simulink model "PID_Cdelta_U"  (R2019b)
settings: Solver=ode4  StartTime=0.0  StopTime=inf  FixedStep=0.05  RelTol=1e-3
InitFcn:
  | initModelParam;
  | SetWaypoints;
values from neighbouring files (symbols this model uses):
  Angsave = zeros(0, WPNum - 1)    [SetWaypoints.m]
  Deltah = 5    [reload.m]
  Deltav = 3    [reload.m]
  P0 = [0,0,0]    [SetWaypoints.m]
  rh = 0.005    [reload.m]
  rv = 0.003    [reload.m]
  Waypoints = [ ... (first row only)    [SetWaypoints.m]
  WPNum = 5    [SetWaypoints.m]
undefined symbols (not defined in the file or in its folder): DiscIntNeverNeededParam
libraries: simulink x3, vrlib x1
settings Model: Creator=53549  LastModifiedBy=51948
settings DataIOCC: ExternalInput=[]  ReturnWorkspaceOutputs=off  OutputSaveName=simOut
settings DebuggingCC: ArithmeticOperatorsInVariantConditions=warning
settings SFSimCC: SimUseLocalCustomCode=off  CustomCodeUndefinedFunction=UseInterfaceOnly
settings RTWCC: RTWUseLocalCustomCode=off
settings CodeAppCC: StateflowObjectComments=on

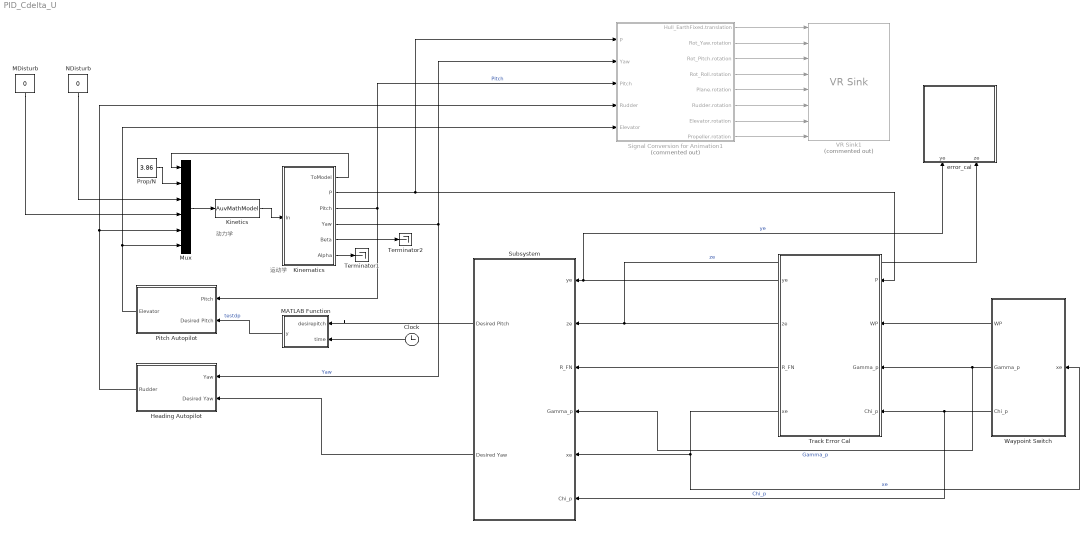
== system PID_Cdelta_U ==
  note: 运动学
  note: 动力学
  Clock : Clock
  Heading Autopilot : Subsystem  mask{kp=2, ki=0, kd=1.5, lambda=0.6, eta=30, epsilon=10, alpha=0.6, Modc=0}
      mask prompts: lambda "滑模表面斜率"; eta "控制增益"; epsilon "防抖动项"; alpha "filter coefficient"; Modc "大于0PID，等于0SMC"
      mask DialogControl DescGroupVar Prompt: Heading Autopilot
      mask DialogControl DescTextVar Prompt: 设置PID增益。
      mask DialogControl ParameterGroupVar Prompt: PID Parameter
  Kinematics : Subsystem  mask{x0=0, y0=0, z0=0.2, pitch0=-10, yaw0=45, u0=0.6, waveAmplitude=[0.2,0.3, 0.05], waveFrequency=[0.1, 0.15,0.2], deR=0.85}
      mask prompts: x0 "Initiral x"; y0 "Initiral y"; z0 "Initiral z"; pitch0 "Initial pitch [Deg]"; yaw0 "Initial yaw [Deg]"; u0 "Initial velocity [m/s]"; deR "decayRate"
      mask init:
      | waveAmplitude = str2num(get_param(gcb, 'waveAmplitude'));
      | waveFrequency = str2num(get_param(gcb, 'waveFrequency'));
      mask DialogControl DescGroupVar Prompt: Kinematics
      mask DialogControl DescTextVar Prompt: Set kinematics information: AMV initial state, flow interference, etc
      mask DialogControl ParameterGroupVar Prompt: Initial state
      mask DialogControl Container3 Prompt: Flow
  Kinetics : MATLABFcn  MATLABFcn=AuvMathModel  OutputDimensions=6  OutputSignalType=real
  MATLAB Function : MATLAB Function  TreatAsAtomicUnit=on
  MDisturb : Constant  Value=0
  Mux : Mux  Inputs=6
  NDisturb : Constant  Value=0
  Pitch Autopilot : Subsystem  mask{kp=3, ki=0.5, kd=1.5, lambda=0.6, eta=30, epsilon=10}
      mask prompts: lambda "滑模表面斜率"; eta "增大控制增益"; epsilon "减小防抖动项"
      mask DialogControl DescGroupVar Prompt: Pitch Autopilot
      mask DialogControl DescTextVar Prompt: 设置PID控制增益。
      mask DialogControl ParameterGroupVar Prompt: PID Parameter
  Prop/N : Constant  Value=3.86
  Signal Conversion for Animation1 : Subsystem  Commented=on
  Subsystem : Subsystem  mask{Deltah=Deltah, Deltav=Deltav, miuc=10, rh=rh, rv=rv}
      mask prompts: Deltah "水平面前视距离"; Deltav "垂直面前视距离"; miuc "极小正常数"; rh "βc自适应增益"; rv "αc自适应增益"
  Terminator1 : Terminator
  Terminator2 : Terminator
  Track Error Cal : MATLAB Function  TreatAsAtomicUnit=on
  VR Sink1 : vrlib/VR Sink  Commented=on  InstantiateOnLoad=on  SampleTime=0.1  ViewEnable=on  RemoteChange=off  RemoteView=off  FieldsWritten=NED.translation.3.1.1.double#RotYaw.rotation.4.1.1.double#RotPitch.rotation.4.1.1.double#RotRoll.rotation.4.1.1.double#Plane.rotation.4.1.1.double#Rudder.rotation.4.1.1.double#Elevator.rotation.4.1.1.double#Rotatation.rotation.4.1.1.double  WorldFileName=SubMarine.wrl  AutoView=on  VideoDimensions=[]  AllowVariableSize=off
      settings: SourceProductName=Simulink
  Waypoint Switch : Subsystem  mask{WP=Waypoints, Angsave=Angsave, WPNum=WPNum}
      mask prompts: WP "航点序列"; Angsave "航点夹角"; WPNum "航点个数"
      mask DialogControl DescGroupVar Prompt: 航点设置
      mask DialogControl DescTextVar Prompt: 设置航点序列和个数
  error_cal : Subsystem
  wires:
  Kinetics/1 -> Kinematics/1(In)
  Mux/1 -> Kinetics/1
  Kinematics/4(Yaw) -> Signal Conversion for Animation1/2(Yaw), Heading Autopilot/1(Yaw)  "Yaw"
  Kinematics/1(ToModel) -> Mux/1
  Prop/N/1 -> Mux/2
  NDisturb/1 -> Mux/3
  Track Error Cal/4(xe) -> Waypoint Switch/1(xe), Subsystem/5(xe)  "xe"
  Waypoint Switch/2(Gamma_p) -> Track Error Cal/3(Gamma_p), Subsystem/4(Gamma_p)  "Gamma_p"
  MDisturb/1 -> Mux/4
  Kinematics/2(P) -> Signal Conversion for Animation1/1(P), Track Error Cal/1(P)
  Kinematics/3(Pitch) -> Signal Conversion for Animation1/3(Pitch), Pitch Autopilot/1(Pitch)  "Pitch"
  Waypoint Switch/3(Chi_p) -> Track Error Cal/4(Chi_p), Subsystem/6(Chi_p)  "Chi_p"
  Waypoint Switch/1(WP) -> Track Error Cal/2(WP)
  Heading Autopilot/1(Rudder) -> Mux/5, Signal Conversion for Animation1/4(Rudder)
  Pitch Autopilot/1(Elevator) -> Signal Conversion for Animation1/5(Elevator), Mux/6
  Signal Conversion for Animation1/1(Hull_EarthFixed.translation) -> VR Sink1/1
  Signal Conversion for Animation1/2(Rot_Yaw.rotation) -> VR Sink1/2
  Signal Conversion for Animation1/3(Rot_Pitch.rotation) -> VR Sink1/3
  Signal Conversion for Animation1/4(Rot_Roll.rotation) -> VR Sink1/4
  Signal Conversion for Animation1/5(Plane.rotation) -> VR Sink1/5
  Signal Conversion for Animation1/8(Propeller.rotation) -> VR Sink1/8
  Signal Conversion for Animation1/6(Rudder.rotation) -> VR Sink1/6
  Signal Conversion for Animation1/7(Elevator.rotation) -> VR Sink1/7
  Subsystem/1(Desired Pitch) -> MATLAB Function/1(desirepitch)
  Subsystem/2(Desired Yaw) -> Heading Autopilot/2(Desired Yaw)
  Track Error Cal/1(ye) -> error_cal/1(ye), Subsystem/1(ye)  "ye"
  Track Error Cal/2(ze) -> error_cal/2(ze), Subsystem/2(ze)  "ze"
  Track Error Cal/3(R_FN) -> Subsystem/3(R_FN)
  Kinematics/6(Alpha) -> Terminator1/1
  Kinematics/5(Beta) -> Terminator2/1
  Clock/1 -> MATLAB Function/2(time)
  MATLAB Function/1(y) -> Pitch Autopilot/2(Desired Pitch)  "testdp"

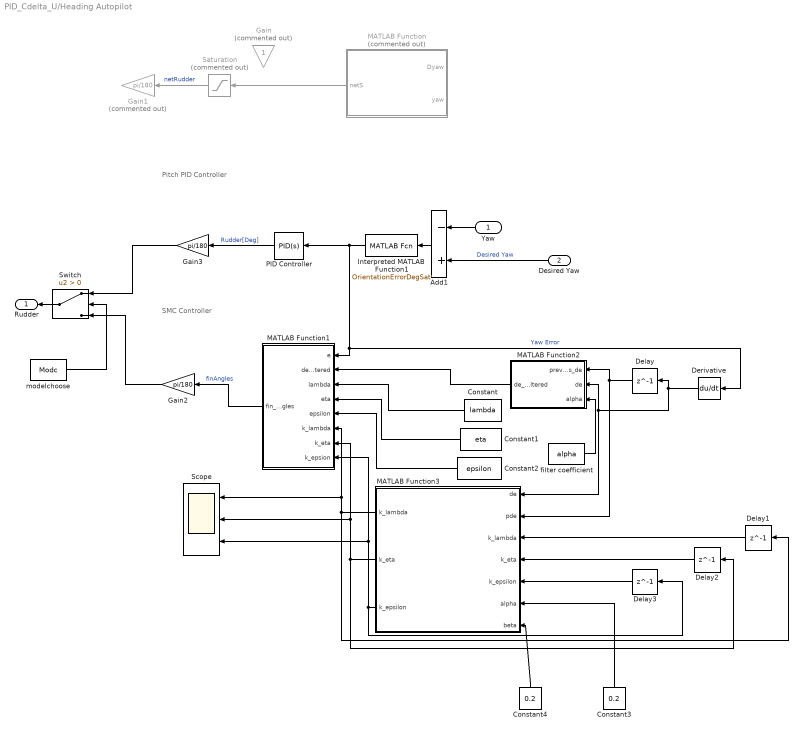
== system PID_Cdelta_U/Heading Autopilot ==
  note: SMC Controller
  note: Pitch PID Controller
  Yaw : Inport
  Desired Yaw : Inport  Port=2
  Add1 : Sum  Inputs=-+
  Constant : Constant  Value=lambda
  Constant1 : Constant  Value=eta
  Constant2 : Constant  Value=epsilon
  Constant3 : Constant  Value=0.2
  Constant4 : Constant  Value=0.2
  Delay{,1..3} (4 alike) : Delay  DelayLength=1
  Derivative : Derivative
  Gain : Gain  Commented=on
  Gain1 : Gain  Commented=on  Gain=pi/180
  Gain2 : Gain  Gain=pi/180
  Gain3 : Gain  Gain=pi/180
  Interpreted MATLAB Function1 : MATLABFcn  MATLABFcn=OrientationErrorDegSat  OutputDimensions=1
  MATLAB Function : MATLAB Function  Commented=on  TreatAsAtomicUnit=on  SystemSampleTime=0.05
  MATLAB Function1 : MATLAB Function  TreatAsAtomicUnit=on
  MATLAB Function2 : MATLAB Function  TreatAsAtomicUnit=on
  MATLAB Function3 : MATLAB Function  TreatAsAtomicUnit=on
  PID Controller : simulink/Continuous/PID Controller  Controller=PID  Form=Parallel  TimeDomain=Continuous-time  SampleTime=-1  IntegratorMethod=Forward Euler  FilterMethod=Forward Euler  ControllerParametersSource=internal  P=kp  I=ki  D=kd  UseFilter=on  N=10  TunerSelectOption=Transfer Function Based (PID Tuner App)  InitialConditionSource=internal  InitialConditionForIntegrator=0  InitialConditionForFilter=0  DifferentiatorICPrevScaledInput=0  ExternalReset=none  TrackingMode=off  Kt=1  LimitOutput=on  UpperSaturationLimit=30  LowerSaturationLimit=-30  LinearizeAsGain=on  AntiWindupMode=none  Kb=1  POutMin=[]  POutMax=[]  IOutMin=[]  IOutMax=[]  DOutMin=[]  DOutMax=[]  NOutMin=[]  NOutMax=[]  SumOutMin=[]  SumOutMax=[]  SaturationOutMin=[]  SaturationOutMax=[]  PParamMin=[]  PParamMax=[]  IParamMin=[]  IParamMax=[]  DParamMin=[]  DParamMax=[]  NParamMin=[]  NParamMax=[]  KbParamMin=[]  KbParamMax=[]  KtParamMin=[]  KtParamMax=[]  KbOutMin=[]  KbOutMax=[]  KtOutMin=[]  KtOutMax=[]  IntegratorOutMin=[]  IntegratorOutMax=[]  FilterOutMin=[]  FilterOutMax=[]  SumI1OutMin=[]  SumI1OutMax=[]  SumI2OutMin=[]  SumI2OutMax=[]  SumI3OutMin=[]  SumI3OutMax=[]  SumI4OutMin=[]  SumI4OutMax=[]  SumDOutMin=[]  SumDOutMax=[]  DifferentiatorOutMin=[]  DifferentiatorOutMax=[]  FilterDiffOutCoefMin=[]  FilterDiffOutCoefMax=[]  ReciprocalOutMin=[]  ReciprocalOutMax=[]  SumDenOutMin=[]  SumDenOutMax=[]  SumNumOutMin=[]  SumNumOutMax=[]  DivideOutMin=[]  DivideOutMax=[]  IntegratorContinuousStateAttributes=''  IntegratorStateMustResolveToSignalObject=off  IntegratorRTWStateStorageClass=Auto  FilterContinuousStateAttributes=''  FilterStateMustResolveToSignalObject=off  FilterRTWStateStorageClass=Auto  ParallelPVariant=InternalParameters  IdealPVariant=Disabled  IVariant=InternalParameters  DVariant=InternalParameters  IntegratorVariant=Continuous  SatVariant=Enabled  AWVariant=Passthrough  PCopyVariant=Disabled  TRVariant=Disabled  FdbkBlocksVariant=Forward  IdealPFdbkVariant=Disabled  SatFdbkVariant=Disabled  DerivativeFilterVariant=ContFilter  NVariant=InternalParameters  NCopyVariant=Disabled  FilterICVariant=InternalICsFilter  IntegratorICVariant=InternalICs  ExternalResetVariant=Disabled  TRSumVariant=Passthrough  SumFdbkVariant=Disabled  SumVariant=Sum_PID
  Saturation : Saturate  Commented=on  UpperLimit=30  LowerLimit=-30
  Scope : Scope  NumInputPorts=3
  Switch : Switch  Criteria=u2 > Threshold
  filter coefficient : Constant  Value=alpha
  modelchoose : Constant  Value=Modc
  Rudder : Outport
  wires:
  Yaw/1 -> Add1/1
  PID Controller/1 -> Gain3/1  "Rudder[Deg]"
  Add1/1 -> Interpreted MATLAB Function1/1
  Desired Yaw/1 -> Add1/2  "Desired Yaw"
  Interpreted MATLAB Function1/1 -> PID Controller/1, Derivative/1, MATLAB Function1/1(e)  "Yaw Error"
  MATLAB Function/1(netS) -> Saturation/1
  Saturation/1 -> Gain1/1  "netRudder"
  MATLAB Function1/1(fin_angles) -> Gain2/1  "finAngles"
  Derivative/1 -> MATLAB Function3/1(de), MATLAB Function2/2(de), Delay/1
  Delay/1 -> MATLAB Function3/2(pde), MATLAB Function2/1(previous_de)
  MATLAB Function2/1(de_filtered) -> MATLAB Function1/2(de_filtered)
  Gain3/1 -> Switch/1
  Constant/1 -> MATLAB Function1/3(lambda)
  Constant1/1 -> MATLAB Function1/4(eta)
  Constant2/1 -> MATLAB Function1/5(epsilon)
  filter coefficient/1 -> MATLAB Function2/3(alpha)
  Switch/1 -> Rudder/1
  Gain2/1 -> Switch/3
  modelchoose/1 -> Switch/2
  MATLAB Function3/1(k_lambda) -> Scope/1, MATLAB Function1/6(k_lambda), Delay1/1
  MATLAB Function3/2(k_eta) -> Scope/2, MATLAB Function1/7(k_eta), Delay2/1
  MATLAB Function3/3(k_epsilon) -> Scope/3, MATLAB Function1/8(k_epsion), Delay3/1
  Constant3/1 -> MATLAB Function3/6(alpha)
  Constant4/1 -> MATLAB Function3/7(beta)
  Delay1/1 -> MATLAB Function3/3("k_lambda ")
  Delay2/1 -> MATLAB Function3/4("k_eta ")
  Delay3/1 -> MATLAB Function3/5("k_epsilon ")

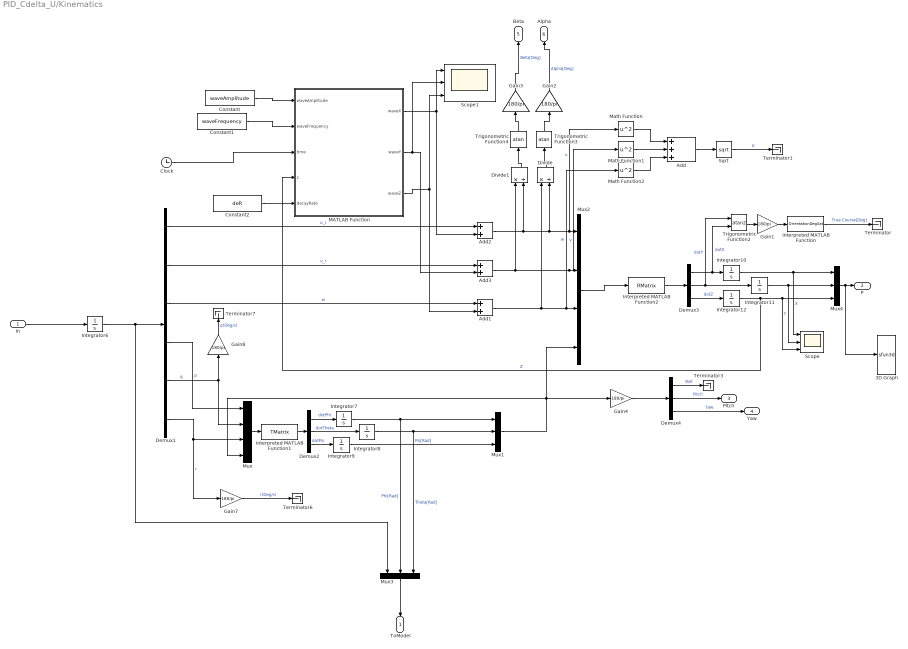
== system PID_Cdelta_U/Kinematics ==
  In : Inport
  3D Graph : S-Function  LoadFcn=if exist('sfun3d','file'), sfun3d([],[],[],'LoadBlock'); end  FunctionName=sfun3d  Parameters=ax,T,np,cp,gd,ls,mk,mx,hd,tb  SFunctionDeploymentMode=off  EnableBusSupport=off  mask(3D Graph){np=1, ax=[-300 300 -300 300 -10 60], mx=1e4, T=0.1, cp=[3 2 1], gd=on, hd=off, tb=off, ls=-, mk=none}
      mask prompts: np "Number of moving points (lines)"; ax "Range: [xmin xmax  ymin ymax zmin zmax]"; mx "Max number of points in each line"; T "Sampling Time"; cp "Camera position (use [0 0 1] for 2D XY view)"; gd "Grid (on|off)"; hd "HeadMarkers (on|off)"; tb "Toolbar (on|off)"; ls "LineStyle"; mk "LineMarker"
      mask help:
      | This block plots the position of several points in the XYZ space. The input contains the coordinates of all the points (x1,y1,z1,x2,y2,z2,...).
      | The number of moving points (lines), the XYZ ranges, sampling time, camera position, and grid (among other things) can be set as mask parameters.
      settings: CopyFcn=if exist('sfun3d','file'), sfun3d([],[],[],'CopyBlock'); end  DeleteFcn=if exist('sfun3d','file'), sfun3d([],[],[],'DeleteBlock'); end  NameChangeFcn=if exist('sfun3d','file'), sfun3d([],[],[],'NameChange'); end
      mask Help:
      | This block plots the position of several points in the XYZ space. The input contains the coordinates of all the points (x1,y1,z1,x2,y2,z2,...).
      | The number of moving points (lines), the XYZ ranges, sampling time, camera position, and grid (among other things) can be set as mask parameters.
      mask TypeOptions ls: - | -- | : | -. | none
      mask TypeOptions mk: none | . | + | o | * | x | square | diamond | v | ^ | > | < | pentagram | hexagram
      mask Display: plot([.05 .95 .95 .05 .05],[.45 .45 .95 .95 .45], 0.5+cos(0:0.1:2*pi)*0.3,0.7+sin(0:0.1:2*pi)*0.2)
  Add : Sum  Inputs=+++
  Add1 : Sum
  Add2 : Sum
  Add3 : Sum
  Clock : Clock
  Constant : Constant  Value=waveAmplitude
  Constant1 : Constant  Value=waveFrequency
  Constant2 : Constant  Value=deR
  Demux1 : Demux  Outputs=6
  Demux2 : Demux  Outputs=3
  Demux3 : Demux  Outputs=3
  Demux4 : Demux  Outputs=3
  Divide : Product  Inputs=*/
  Divide1 : Product  Inputs=*/
  Gain{1..4,7..8} (6 alike) : Gain  Gain=180/pi
  Integrator10 : Integrator  InitialCondition=x0
  Integrator11 : Integrator  InitialCondition=y0
  Integrator12 : Integrator  InitialCondition=z0
  Integrator6 : Integrator  InitialCondition=[u0; 0; 0; 0; 0; 0]
  Integrator7 : Integrator
  Integrator8 : Integrator  InitialCondition=pitch0/180*pi
  Integrator9 : Integrator  InitialCondition=yaw0*pi/180  WrapState=on  WrappedStateUpperValue=6.2832  WrappedStateLowerValue=0
  Interpreted MATLAB Function : MATLABFcn  MATLABFcn=OrientationDegSat
  Interpreted MATLAB Function1 : MATLABFcn  MATLABFcn=TMatrix  OutputDimensions=3
  Interpreted MATLAB Function2 : MATLABFcn  MATLABFcn=RMatrix  OutputDimensions=3
  MATLAB Function : MATLAB Function  TreatAsAtomicUnit=on
  Math Function : Math  Operator=square  SignedPower=off  SaturateOnIntegerOverflow=on
  Math Function1 : Math  Operator=square  SignedPower=off  SaturateOnIntegerOverflow=on
  Math Function2 : Math  Operator=square  SignedPower=off  SaturateOnIntegerOverflow=on
  Mux : Mux
  Mux1 : Mux  Inputs=3
  Mux2 : Mux
  Mux3 : Mux  Inputs=3
  Mux4 : Mux  Inputs=3
  Scope : Scope  NumInputPorts=3
  Scope1 : Scope  NumInputPorts=3
  Sqrt : Sqrt  SaturateOnIntegerOverflow=on
  Terminator{,1,3,6..7} (5 alike) : Terminator
  Trigonometric Function2 : Trigonometry  Operator=atan2
  Trigonometric Function3 : Trigonometry  Operator=atan
  Trigonometric Function4 : Trigonometry  Operator=atan
  ToModel : Outport
  P : Outport  Port=2
  Pitch : Outport  Port=3
  Yaw : Outport  Port=4
  Beta : Outport  Port=5
  Alpha : Outport  Port=6
  wires:
  Integrator6/1 -> Demux1/1, Mux3/1
  Demux1/4 -> Mux/1  "p"
  Demux1/5 -> Mux/2, Gain8/1  "q"
  Demux1/6 -> Mux/3, Gain7/1  "r"
  Mux/1 -> Interpreted MATLAB Function1/1
  Interpreted MATLAB Function1/1 -> Demux2/1
  Demux2/1 -> Integrator7/1  "dotPhi"
  Demux2/2 -> Integrator8/1  "dotTheta"
  Demux2/3 -> Integrator9/1  "dotPsi"
  Integrator9/1 -> Mux1/3  "Psi[Rad]"
  Integrator7/1 -> Mux1/1, Mux3/2  "Phi[Rad]"
  Integrator8/1 -> Mux1/2, Mux3/3  "Theta[Rad]"
  Mux1/1 -> Gain4/1, Mux/4, Mux2/4
  Demux1/1 -> Add2/1  "u_r"
  Demux1/2 -> Add3/1  "v_r"
  Demux1/3 -> Add1/1  "w"
  Mux2/1 -> Interpreted MATLAB Function2/1
  Interpreted MATLAB Function2/1 -> Demux3/1
  Demux3/1 -> Trigonometric Function2/2, Integrator10/1  "dotX"
  Demux3/2 -> Trigonometric Function2/1, Integrator11/1  "dotY"
  Demux3/3 -> Integrator12/1  "dotZ"
  Integrator10/1 -> Scope/1, Mux4/1  "X"
  Integrator11/1 -> Mux4/2, Scope/2  "Y"
  Integrator12/1 -> MATLAB Function/4(z), Mux4/3, Scope/3  "Z"
  Gain2/1 -> Alpha/1  "Alpha[Deg]"
  Trigonometric Function3/1 -> Gain2/1
  Divide/1 -> Trigonometric Function3/1
  Divide1/1 -> Trigonometric Function4/1
  Trigonometric Function4/1 -> Gain3/1
  Gain3/1 -> Beta/1  "Beta[Deg]"
  Gain1/1 -> Interpreted MATLAB Function/1
  Interpreted MATLAB Function/1 -> Terminator/1  "True Course[Deg]"
  Trigonometric Function2/1 -> Gain1/1
  Add2/1 -> Math Function/1, Mux2/1, Divide/2, Divide1/2  "u"
  Add3/1 -> Math Function1/1, Mux2/2, Divide1/1  "v"
  Gain4/1 -> Demux4/1
  Demux4/1 -> Terminator3/1  "Roll"
  Demux4/2 -> Pitch/1  "Pitch"
  Demux4/3 -> Yaw/1  "Yaw"
  Mux3/1 -> ToModel/1
  Mux4/1 -> 3D Graph/1, P/1
  In/1 -> Integrator6/1
  Gain7/1 -> Terminator6/1  "r(Deg/s)"
  Gain8/1 -> Terminator7/1  "q(Deg/s)"
  Constant/1 -> MATLAB Function/1(waveAmplitude)
  Constant1/1 -> MATLAB Function/2(waveFrequency)
  Constant2/1 -> MATLAB Function/5(decayRate)
  Add1/1 -> Mux2/3, Math Function2/1, Divide/1  "w"
  MATLAB Function/2(waveY) -> Add3/2, Scope1/2
  MATLAB Function/3(waveZ) -> Add1/2, Scope1/3
  Clock/1 -> MATLAB Function/3(time)
  MATLAB Function/1(waveX) -> Add2/2, Scope1/1
  Math Function1/1 -> Add/2
  Math Function/1 -> Add/1
  Math Function2/1 -> Add/3
  Add/1 -> Sqrt/1
  Sqrt/1 -> Terminator1/1  "U"

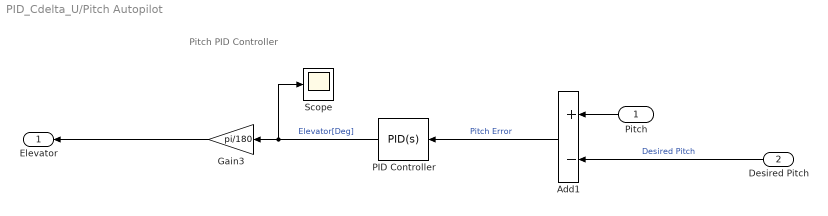
== system PID_Cdelta_U/Pitch Autopilot ==
  note: Pitch PID Controller
  Pitch : Inport
  Desired Pitch : Inport  Port=2
  Add1 : Sum  Inputs=+-
  Gain3 : Gain  Gain=pi/180
  PID Controller : simulink/Continuous/PID Controller  Controller=PID  Form=Parallel  TimeDomain=Continuous-time  SampleTime=-1  IntegratorMethod=Forward Euler  FilterMethod=Forward Euler  ControllerParametersSource=internal  P=kp  I=ki  D=kd  UseFilter=on  N=10  TunerSelectOption=Transfer Function Based (PID Tuner App)  InitialConditionSource=internal  InitialConditionForIntegrator=0  InitialConditionForFilter=0  DifferentiatorICPrevScaledInput=0  ExternalReset=none  TrackingMode=off  Kt=1  LimitOutput=on  UpperSaturationLimit=30  LowerSaturationLimit=-30  LinearizeAsGain=on  AntiWindupMode=none  Kb=1  POutMin=[]  POutMax=[]  IOutMin=[]  IOutMax=[]  DOutMin=[]  DOutMax=[]  NOutMin=[]  NOutMax=[]  SumOutMin=[]  SumOutMax=[]  SaturationOutMin=[]  SaturationOutMax=[]  PParamMin=[]  PParamMax=[]  IParamMin=[]  IParamMax=[]  DParamMin=[]  DParamMax=[]  NParamMin=[]  NParamMax=[]  KbParamMin=[]  KbParamMax=[]  KtParamMin=[]  KtParamMax=[]  KbOutMin=[]  KbOutMax=[]  KtOutMin=[]  KtOutMax=[]  IntegratorOutMin=[]  IntegratorOutMax=[]  FilterOutMin=[]  FilterOutMax=[]  SumI1OutMin=[]  SumI1OutMax=[]  SumI2OutMin=[]  SumI2OutMax=[]  SumI3OutMin=[]  SumI3OutMax=[]  SumI4OutMin=[]  SumI4OutMax=[]  SumDOutMin=[]  SumDOutMax=[]  DifferentiatorOutMin=[]  DifferentiatorOutMax=[]  FilterDiffOutCoefMin=[]  FilterDiffOutCoefMax=[]  ReciprocalOutMin=[]  ReciprocalOutMax=[]  SumDenOutMin=[]  SumDenOutMax=[]  SumNumOutMin=[]  SumNumOutMax=[]  DivideOutMin=[]  DivideOutMax=[]  IntegratorContinuousStateAttributes=''  IntegratorStateMustResolveToSignalObject=off  IntegratorRTWStateStorageClass=Auto  FilterContinuousStateAttributes=''  FilterStateMustResolveToSignalObject=off  FilterRTWStateStorageClass=Auto  ParallelPVariant=InternalParameters  IdealPVariant=Disabled  IVariant=InternalParameters  DVariant=InternalParameters  IntegratorVariant=Continuous  SatVariant=Enabled  AWVariant=Passthrough  PCopyVariant=Disabled  TRVariant=Disabled  FdbkBlocksVariant=Forward  IdealPFdbkVariant=Disabled  SatFdbkVariant=Disabled  DerivativeFilterVariant=ContFilter  NVariant=InternalParameters  NCopyVariant=Disabled  FilterICVariant=InternalICsFilter  IntegratorICVariant=InternalICs  ExternalResetVariant=Disabled  TRSumVariant=Passthrough  SumFdbkVariant=Disabled  SumVariant=Sum_PID
  Scope : Scope
  Elevator : Outport
  wires:
  Add1/1 -> PID Controller/1  "Pitch Error"
  PID Controller/1 -> Scope/1, Gain3/1  "Elevator[Deg]"
  Pitch/1 -> Add1/1
  Gain3/1 -> Elevator/1
  Desired Pitch/1 -> Add1/2  "Desired Pitch"

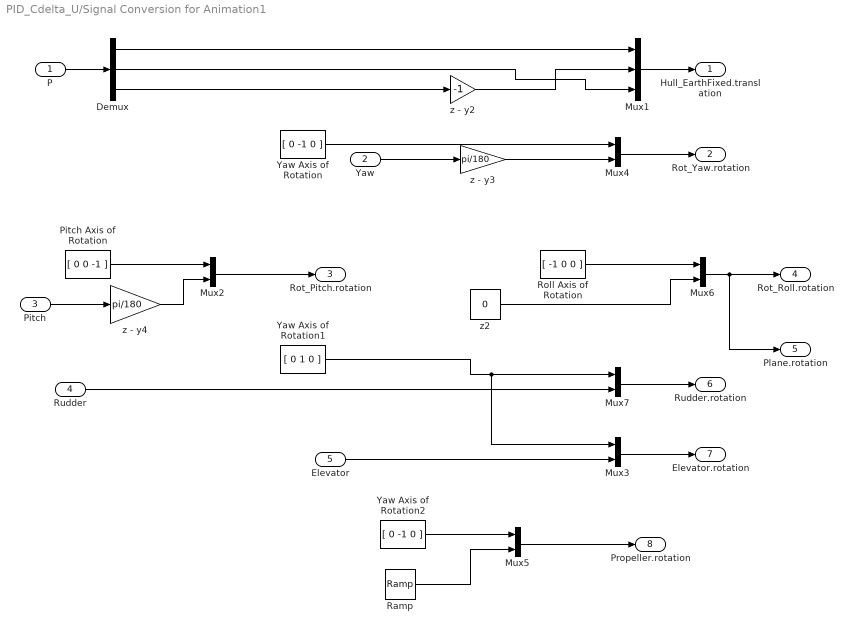
== system PID_Cdelta_U/Signal Conversion for Animation1 ==
  P : Inport
  Yaw : Inport  Port=2
  Pitch : Inport  Port=3
  Rudder : Inport  Port=4
  Elevator : Inport  Port=5
  Demux : Demux  Outputs=3
  Mux1 : Mux  Inputs=3
  Mux{2..7} (6 alike) : Mux  Inputs=2
  Pitch Axis of Rotation : Constant  Value=[ 0 0 -1 ]
  Ramp : simulink/Sources/Ramp  slope=2  start=0  InitialOutput=0
  Roll Axis of Rotation : Constant  Value=[ -1 0 0 ]
  Yaw Axis of Rotation : Constant  Value=[ 0 -1 0 ]
  Yaw Axis of Rotation1 : Constant  Value=[ 0 1 0 ]
  Yaw Axis of Rotation2 : Constant  Value=[ 0 -1 0 ]
  z - y2 : Gain  Gain=-1
  z - y3 : Gain  Gain=pi/180
  z - y4 : Gain  Gain=pi/180
  z2 : Constant  Value=0
  Hull_EarthFixed.translation : Outport
  Rot_Yaw.rotation : Outport  Port=2
  Rot_Pitch.rotation : Outport  Port=3
  Rot_Roll.rotation : Outport  Port=4
  Plane.rotation : Outport  Port=5
  Rudder.rotation : Outport  Port=6
  Elevator.rotation : Outport  Port=7
  Propeller.rotation : Outport  Port=8
  wires:
  Roll Axis of Rotation/1 -> Mux6/1
  z2/1 -> Mux6/2
  Demux/3 -> z - y2/1
  z - y2/1 -> Mux1/2
  Demux/2 -> Mux1/3
  Yaw Axis of Rotation/1 -> Mux4/1
  Mux1/1 -> Hull_EarthFixed.translation/1
  P/1 -> Demux/1
  Rudder/1 -> Mux7/2
  Mux7/1 -> Rudder.rotation/1
  Mux4/1 -> Rot_Yaw.rotation/1
  Mux6/1 -> Plane.rotation/1, Rot_Roll.rotation/1
  Yaw/1 -> z - y3/1
  Pitch Axis of Rotation/1 -> Mux2/1
  Mux2/1 -> Rot_Pitch.rotation/1
  z - y4/1 -> Mux2/2
  Pitch/1 -> z - y4/1
  Demux/1 -> Mux1/1
  z - y3/1 -> Mux4/2
  Yaw Axis of Rotation1/1 -> Mux3/1, Mux7/1
  Mux3/1 -> Elevator.rotation/1
  Elevator/1 -> Mux3/2
  Yaw Axis of Rotation2/1 -> Mux5/1
  Mux5/1 -> Propeller.rotation/1
  Ramp/1 -> Mux5/2

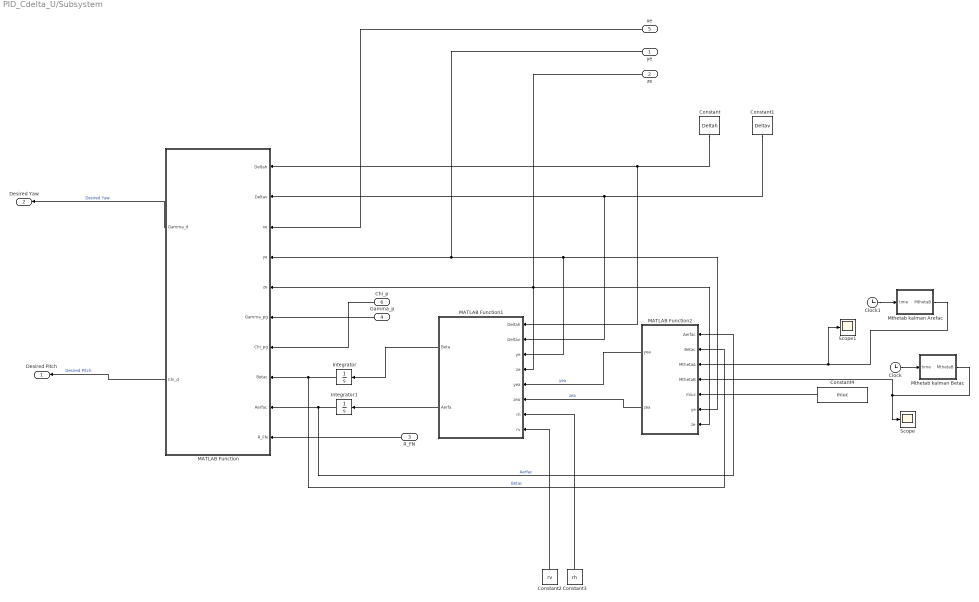
== system PID_Cdelta_U/Subsystem ==
  ye : Inport
  ze : Inport  Port=2
  R_FN : Inport  Port=3
  Gamma_p : Inport  Port=4
  xe : Inport  Port=5
  Chi_p : Inport  Port=6
  Clock : Clock
  Clock1 : Clock
  Constant : Constant  Value=Deltah
  Constant1 : Constant  Value=Deltav
  Constant2 : Constant  Value=rv
  Constant3 : Constant  Value=rh
  Constant4 : Constant  Value=miuc
  Integrator : Integrator
  Integrator1 : Integrator
  MATLAB Function : MATLAB Function  TreatAsAtomicUnit=on
  MATLAB Function1 : MATLAB Function  TreatAsAtomicUnit=on
  MATLAB Function2 : MATLAB Function  TreatAsAtomicUnit=on
  Mthetab kalman Arefac : MATLAB Function  TreatAsAtomicUnit=on  SystemSampleTime=0.05
  "Mthetab kalman Betac " : MATLAB Function  TreatAsAtomicUnit=on  SystemSampleTime=0.05
  Scope : Scope
  Scope1 : Scope
  Desired Pitch : Outport
  Desired Yaw : Outport  Port=2
  wires:
  ze/1 -> MATLAB Function1/4(ze), MATLAB Function2/7(ze), MATLAB Function/5(ze)
  Integrator1/1 -> MATLAB Function/9(Aerfac), MATLAB Function2/1(Aerfac)  "Aerfac"
  Constant2/1 -> MATLAB Function1/8(rv)
  Constant/1 -> MATLAB Function/1(Deltah), MATLAB Function1/1(Deltah)
  Constant1/1 -> MATLAB Function/2(Deltav), MATLAB Function1/2(Deltav)
  ye/1 -> MATLAB Function1/3(ye), MATLAB Function2/6(ye), MATLAB Function/4(ye)
  MATLAB Function1/1(Beta) -> Integrator/1
  Constant3/1 -> MATLAB Function1/7(rh)
  Integrator/1 -> MATLAB Function2/2(Betac), MATLAB Function/8(Betac)  "Betac"
  MATLAB Function1/2(Aerfa) -> Integrator1/1
  MATLAB Function/2(Chi_d) -> Desired Pitch/1  "Desired Pitch"
  R_FN/1 -> MATLAB Function/10(R_FN)
  Chi_p/1 -> MATLAB Function/7(Chi_pg)
  Gamma_p/1 -> MATLAB Function/6(Gamma_pg)
  xe/1 -> MATLAB Function/3(xe)
  MATLAB Function/1(Gamma_d) -> Desired Yaw/1  "Desired Yaw"
  MATLAB Function2/1(yea) -> MATLAB Function1/5(yea)  "yea"
  MATLAB Function2/2(zea) -> MATLAB Function1/6(zea)  "zea"
  Constant4/1 -> MATLAB Function2/5(miuc)
  Mthetab kalman Arefac/1(MthetaB) -> MATLAB Function2/3(MthetaA), Scope1/1
  "Mthetab kalman Betac "/1(MthetaB) -> Scope/1, MATLAB Function2/4(MthetaB)
  Clock/1 -> "Mthetab kalman Betac "/1(time)
  Clock1/1 -> Mthetab kalman Arefac/1(time)

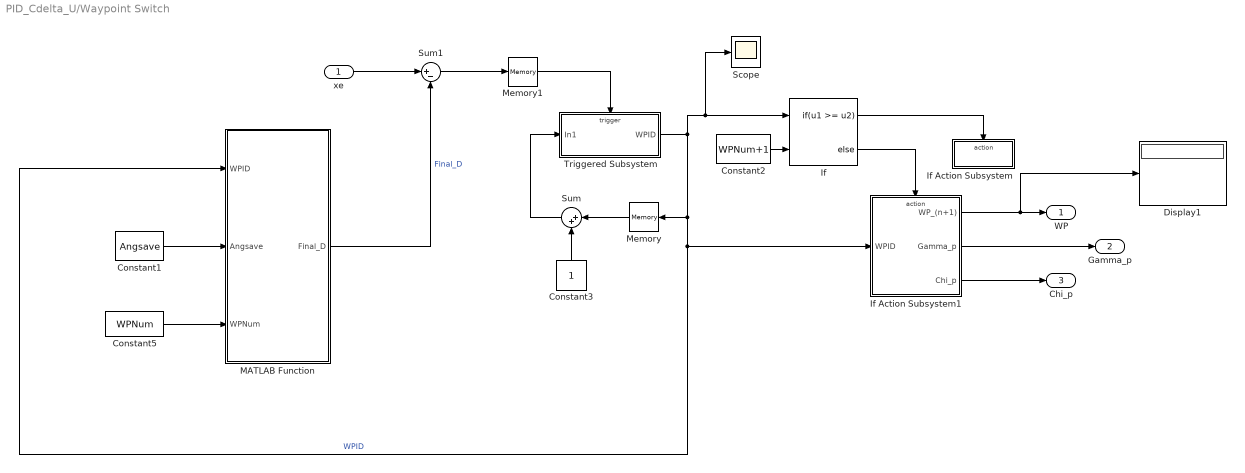
== system PID_Cdelta_U/Waypoint Switch ==
  xe : Inport
  Constant1 : Constant  Value=Angsave
  Constant2 : Constant  Value=WPNum+1
  Constant3 : Constant
  Constant5 : Constant  Value=WPNum
  Display1 : Display
  If : If  NumInputs=2  IfExpression=u1 >= u2
  If Action Subsystem : Subsystem  TreatAsAtomicUnit=on
  If Action Subsystem1 : Subsystem  TreatAsAtomicUnit=on
  MATLAB Function : MATLAB Function  TreatAsAtomicUnit=on
  Memory : Memory  InitialCondition=1  InheritSampleTime=on
  Memory1 : Memory  InitialCondition=5  InheritSampleTime=on
  Scope : Scope
  Sum : Sum  Inputs=|++
  Sum1 : Sum  Inputs=|+-
  Triggered Subsystem : Subsystem  TreatAsAtomicUnit=on
  WP : Outport
  Gamma_p : Outport  Port=2
  Chi_p : Outport  Port=3
  wires:
  Constant2/1 -> If/2
  If Action Subsystem1/2(Gamma_p) -> Gamma_p/1
  Sum1/1 -> Memory1/1
  Memory/1 -> Sum/1
  If/2 -> If Action Subsystem1/Action
  xe/1 -> Sum1/1
  Sum/1 -> Triggered Subsystem/1(In1)
  Constant3/1 -> Sum/2
  If Action Subsystem1/1(WP_(n+1)) -> Display1/1, WP/1
  Triggered Subsystem/1(WPID) -> MATLAB Function/1(WPID), If Action Subsystem1/1(WPID), Memory/1, Scope/1, If/1  "WPID"
  If/1 -> If Action Subsystem/Action
  Memory1/1 -> Triggered Subsystem/Trigger
  If Action Subsystem1/3(Chi_p) -> Chi_p/1
  MATLAB Function/1(Final_D) -> Sum1/2  "Final_D"
  Constant1/1 -> MATLAB Function/2(Angsave)
  Constant5/1 -> MATLAB Function/3(WPNum)

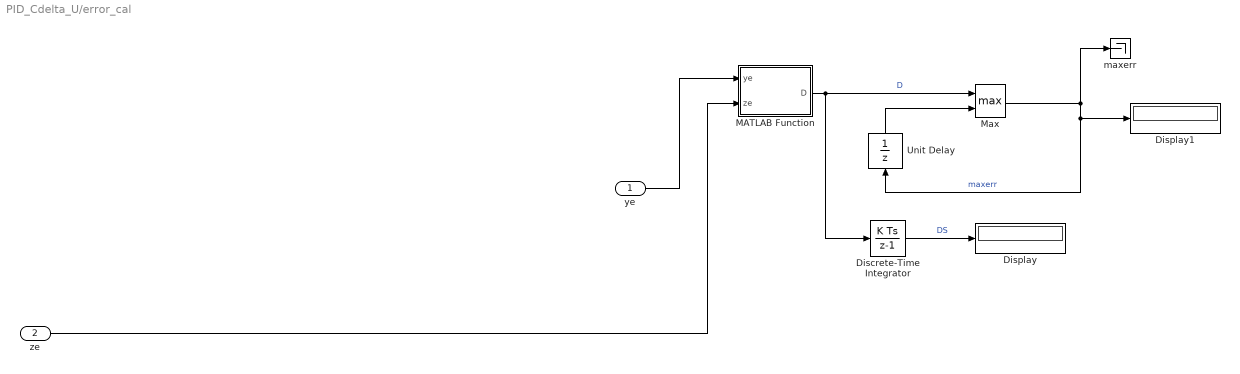
== system PID_Cdelta_U/error_cal ==
  ye : Inport
  ze : Inport  Port=2
  Discrete-Time Integrator : DiscreteIntegrator  SampleTime=-1  ICPrevOutput=DiscIntNeverNeededParam  ICPrevScaledInput=DiscIntNeverNeededParam
  Display : Display
  Display1 : Display
  MATLAB Function : MATLAB Function  TreatAsAtomicUnit=on
  Max : MinMax  Function=max  Inputs=2
  Unit Delay : UnitDelay  SampleTime=-1  HasFrameUpgradeWarning=on
  maxerr : Terminator
  wires:
  ye/1 -> MATLAB Function/1(ye)
  Max/1 -> maxerr/1, Unit Delay/1, Display1/1  "maxerr"
  ze/1 -> MATLAB Function/2(ze)
  Unit Delay/1 -> Max/2
  Discrete-Time Integrator/1 -> Display/1  "DS"
  MATLAB Function/1(D) -> Discrete-Time Integrator/1, Max/1  "D"

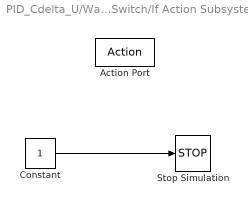
== system PID_Cdelta_U/Waypoint Switch/If Action Subsystem ==
  Action Port : ActionPort  ActionPortLabel=if(u1 >= u2)
  Constant : Constant
  Stop Simulation : Stop
  wires:
  Constant/1 -> Stop Simulation/1

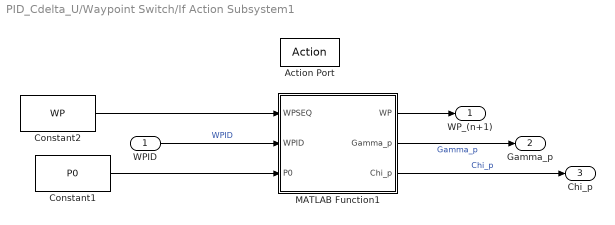
== system PID_Cdelta_U/Waypoint Switch/If Action Subsystem1 ==
  WPID : Inport
  Action Port : ActionPort  ActionPortLabel=else
  Constant1 : Constant  Value=P0
  Constant2 : Constant  Value=WP
  MATLAB Function1 : MATLAB Function  TreatAsAtomicUnit=on
  WP_(n+1) : Outport
  Gamma_p : Outport  Port=2
  Chi_p : Outport  Port=3
  wires:
  MATLAB Function1/2(Gamma_p) -> Gamma_p/1  "Gamma_p"
  MATLAB Function1/1(WP) -> WP_(n+1)/1
  Constant2/1 -> MATLAB Function1/1(WPSEQ)
  WPID/1 -> MATLAB Function1/2(WPID)  "WPID"
  MATLAB Function1/3(Chi_p) -> Chi_p/1  "Chi_p"
  Constant1/1 -> MATLAB Function1/3(P0)

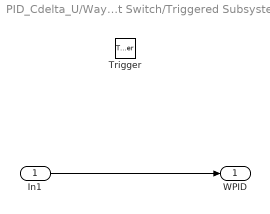
== system PID_Cdelta_U/Waypoint Switch/Triggered Subsystem ==
  In1 : Inport
  Trigger : TriggerPort  TriggerType=falling  VariantControl=Variant
  WPID : Outport  InitialOutput=1
  wires:
  In1/1 -> WPID/1

== matlab function PID_Cdelta_U/Waypoint Switch/If Action Subsystem1/MATLAB Function1 ==
  data: WP output; WPSEQ input; WPID input; Gamma_p output; Chi_p output; P0 input
function [WP,Gamma_p,Chi_p] = fcn(WPSEQ,WPID,P0)
WP = WPSEQ(WPID,:)';

if WPID == 1
    dx = WPSEQ(1,1)-P0(1);dy = WPSEQ(1,2)-P0(2);dz = WPSEQ(1,3)-P0(3);
else
    dp = WPSEQ(WPID,:)-WPSEQ(WPID-1,:);
    dx = dp(1);dy = dp(2);dz = dp(3);
end

Gamma_p = atan2(dy,dx);
Chi_p = atan2(-dz,sqrt(dx*dx+dy*dy));

if Gamma_p<0
    Gamma_p = Gamma_p + 2*pi;
end
    
end

== matlab function PID_Cdelta_U/Track Error Cal ==
  data: ye output; ze output; P input; WP input; Gamma_p input; Chi_p input; R_FN output; xe output
function [ye,ze,R_FN,xe] = fcn(P,WP,Gamma_p,Chi_p)                      
sg = sin(Gamma_p);cg = cos(Gamma_p);
sc = sin(Chi_p);cc = cos(Chi_p);
R_FN = [cg*cc -sg cg*sc; 
            sg*cc cg sg*sc;
                -sc 0 cc];
R_NF = R_FN';
E_F = R_NF*(WP-P);

xe = E_F(1);
ye = E_F(2);
ze = E_F(3);
end


% Gamma_p -- Xp/pih
% Chi_p -- vp/piv
% R_FN -- Rp =Rpx*Rpv(37)
% WP -- p
% P -- pp(w)
% E_F -- 误差矩阵(38)

== matlab function PID_Cdelta_U/Kinematics/MATLAB Function ==
  data: waveAmplitude input; waveFrequency input; waveX output size=1; time input; z input; decayRate input; waveY output; waveZ output
function [waveX, waveY, waveZ] = simulateWaveEffect3D(waveAmplitude, waveFrequency, time, z, decayRate)
    % velocity0: 初始速度，单位 [m/s]，向量 [vx0, vy0, vz0]
    % waveAmplitude: 海浪振幅，单位 [m]，向量 [ax, ay, az]
    % waveFrequency: 海浪频率，单位 [Hz]，向量 [fx, fy, fz]
    % time: 仿真时间，单位 s
    % depth: 水下机器人的深度，单位 m
    % decayRate: 海浪影响随深度衰减的速率，推荐值为 0.5 到 1.0

    
    % 时间步长
    %dt = 0.05;
    %t = 0:dt:time; % 仿真时间范围，步长为0.05秒

    % 计算每个方向的海浪影响，考虑深度衰减
    waveX = waveAmplitude(1) * exp(-decayRate * z) * sin(2 * pi * waveFrequency(1) * time);
    waveY = waveAmplitude(2) * exp(-decayRate * z) * sin(2 * pi * waveFrequency(2) * time);
    waveZ = waveAmplitude(3) * exp(-decayRate * z) * sin(2 * pi * waveFrequency(3) * time);

%     % 绘制速度随时间的变化曲线
%     figure;
%     subplot(3,1,1);
%     plot(t, velocityX);
%     xlabel('Time (s)');
%     ylabel('Velocity X (m/s)');
%     title('Velocity X of Underwater Robot under Wave Effect');
%     grid on;
% 
%     subplot(3,1,2);
%     plot(t, velocityY);
%     xlabel('Time (s)');
%     ylabel('Velocity Y (m/s)');
%     title('Velocity Y of Underwater Robot under Wave Effect');
%     grid on;
% 
%     subplot(3,1,3);
%     plot(t, velocityZ);
%     xlabel('Time (s)');
%     ylabel('Velocity Z (m/s)');
%     title('Velocity Z of Underwater Robot under Wave Effect');
%     grid on;
end

== matlab function PID_Cdelta_U/Subsystem/MATLAB Function ==
  data: Deltah input; Gamma_d output; Deltav input; xe input; ye input; ze input; Gamma_pg input; Chi_pg input; Betac input; Aerfac input; Chi_d output; R_FN input
function [Gamma_d,Chi_d]   = fcn(Deltah,Deltav,xe,ye,ze,Gamma_pg,Chi_pg,Betac,Aerfac,R_FN)

LOS_F = [xe;ye;ze];      %误差矩阵
LOS_N = R_FN*LOS_F;

% yea = LOS_N(2)
% zea = LOS_N(3);
%Gamma_d =  Gamma_pg - Betac - atan(LOS_N(2)/Deltah);
% Gamma_d = atan2(LOS_N(3),Deltah) +Betac ;
%Gamma_d = atan2(LOS_N(2),sign(LOS_N(1))*sqrt(LOS_N(1)*LOS_N(1)+LOS_N(3)*LOS_N(3)));
Gamma_d =  Gamma_pg + Betac + atan(LOS_F(2)/Deltah);

% Gamma_d = Gamma_d*180/pi;

 Chi_d = - ( - Chi_pg + Aerfac + atan(LOS_F(3)/Deltav))  * 180 / pi;
% Chi_d = (-atan(LOS_N(3)/sqrt(Deltav^2+LOS_N(2)^2)) - Aerfac)*180/pi;
%Chi_d = -atan(LOS_N(3)/abs(LOS_N(1)))*180/pi;

if Gamma_d<0
    Gamma_d = Gamma_d+2*pi;
end

Gamma_d = Gamma_d*180/pi;


end

== matlab function PID_Cdelta_U/Subsystem/MATLAB Function1 ==
  data: Deltah input; Beta output; Deltav input; ye input; ze input; yea input; zea input; rh input; rv input; Aerfa output
function [Beta,Aerfa] = fcn(Deltah,Deltav,ye,ze,yea,zea,rh,rv)

Beta = rh * (Deltah / sqrt(Deltah^2 + ye^2)) * yea;
Aerfa = rv * (Deltav / sqrt(Deltav^2 + ze^2)) * zea;

end

== matlab function PID_Cdelta_U/Subsystem/MATLAB Function2 ==
  data: Aerfac input; yea output; Betac input; MthetaA input; MthetaB input; miuc input; ye input; ze input; zea output
function [yea, zea] = fcn(Aerfac, Betac,MthetaA, MthetaB, miuc, ye, ze)

if (abs(Betac) > MthetaB) && (Betac * ye > 0)
    yea = (1 - min(1, (Betac^2 - MthetaB^2)/((MthetaB + miuc)^2 - MthetaB^2)))*ye;
else
    yea = ye;
end

if (abs(Aerfac) > MthetaA) && (Aerfac * ze > 0)
    zea = (1 - min(1, (Aerfac^2 - MthetaA^2)/((MthetaA + miuc)^2 - MthetaA^2)))*ze;
else
    zea = ze;
end



end

== matlab function PID_Cdelta_U/error_cal/MATLAB Function ==
  data: ye input; D output; ze input
function D = fcn(ye, ze)

D = sqrt(ye^2 + ze^2);

end

== matlab function PID_Cdelta_U/Subsystem/Mthetab kalman Betac  ==
  data: time input; MthetaB output
function MthetaB = b(time)
%#codegen

t = time/0.05;

persistent x_saved y_saved  % 声明持久变量

if isempty(x_saved) || isempty(y_saved)
    % 加载保存的数据，仅在第一次调用时执行
    data = load('databc.mat', 't', 'y');
    x_saved = data.t;
    y_saved = data.y;
end

% 查询数据
MthetaB = interp1(x_saved, y_saved, t, 'linear', 'extrap');
end

== matlab function PID_Cdelta_U/MATLAB Function ==
  data: desirepitch input; y output; time input
function y = fcn(desirepitch, time)

    if time >=0 && time<=5
        y = desirepitch + 2.3 * time  - 11.5;
    else
        y = desirepitch;
    end


end

== matlab function PID_Cdelta_U/Subsystem/Mthetab kalman Arefac ==
  data: time input; MthetaB output
function MthetaB = b(time)
%#codegen

t = time/0.05;

persistent x_saved y_saved  % 声明持久变量

if isempty(x_saved) || isempty(y_saved)
    % 加载保存的数据，仅在第一次调用时执行
    data = load('dataac.mat', 't', 'y');
    x_saved = data.t;
    y_saved = data.y;
end

% 查询数据
MthetaB = interp1(x_saved, y_saved, t, 'linear', 'extrap');
end

== matlab function PID_Cdelta_U/Waypoint Switch/MATLAB Function ==
  data: WPID input; Final_D output; Angsave input; WPNum input
function Final_D = cal_acceptD(WPID, Angsave, WPNum)

    if WPID <= WPNum -1
        Final_D = 11.1463 * Angsave(WPID) - 3.2553;
    else
        Final_D = 11.1463 * Angsave(WPID -2) - 3.2553;
    end

end

== matlab function PID_Cdelta_U/Heading Autopilot/MATLAB Function ==
  data: netS output; Dyaw input; yaw input
function netS = predictKA(Dyaw, yaw)
%     % 加载训练好的模型
    persistent fnB fnT;
    if isempty(fnB) || isempty(fnT)
        data = load('trainedKAmodel.mat');
        fnB = data.fnB;
        fnT = data.fnT;
    end
    
   
    
    
%     m = 6;
%     x = rand(1,m);
    
    % 输入数据归一化（根据训练时的数据范围调整）
    xmin = 0; xmax = 360;
    ymin = -30; ymax = 30;
%     
    % 创建一个 3x3 的矩阵
%     dd = zeros(1, 6);  % 初始化为零矩阵
    

    dd = [yaw Dyaw];



    netS = Copy_of_modelKA_basisC(dd, xmin, xmax, ymin, ymax, fnB, fnT );

    



  
end

== matlab function PID_Cdelta_U/Heading Autopilot/MATLAB Function1 ==
  data: e input; fin_angles output; de_filtered input; lambda input; eta input; epsilon input; k_lambda input; k_eta input; k_epsion input
function fin_angles = fcn(e, de_filtered, lambda, eta, epsilon, k_lambda, k_eta, k_epsion )
    
    % lambda = 0.6;     % 增大滑模表面斜率
    % eta = 30.0;        % 增大控制增益
    % epsilon = 10;  % 减小防抖动项
    
    lambda  =  lambda + lambda * k_lambda;
    eta = eta + eta * k_eta;
    epsilon = epsilon + epsilon * k_epsion;

    s = lambda * e + de_filtered;
    
    % 自适应滑模控制律
    if abs(s) > epsilon
        % 当滑模面绝对值大于防抖动项时，使用标准滑模控制律
        fin_angles = eta * sign(s);
    else
        % 当滑模面绝对值小于防抖动项时，使用平滑控制
        fin_angles = eta * s / epsilon;
    end
    

    
    
end

== matlab function PID_Cdelta_U/Heading Autopilot/MATLAB Function2 ==
  data: previous_de input; de_filtered output; de input; alpha input
function de_filtered = fcn(previous_de, de, alpha)


% 滤波器系数保持不变
% alpha = 0.6;     

% 假设有上次的误差导数存储
%   previous_dein = 0;  

% 计算误差导数并进行滤波
de_filtered = alpha * de + (1 - alpha) * previous_de;



end

== matlab function PID_Cdelta_U/Heading Autopilot/MATLAB Function3 ==
  data: de input; k_lambda output; pde input; k_eta output; k_epsilon output; k_lambda input; k_eta input; k_epsilon input; alpha input; beta input
function [k_lambda, k_eta, k_epsilon] = adaptive_control( de, pde, k_lambda, k_eta, k_epsilon, alpha, beta)
    % 参数初始化
    delta_de = de - pde; % 误差导数的变化量
    
    % 自适应调整k_lambda
    if delta_de < 0 % 如果误差在减小
        k_lambda = k_lambda * (1 - alpha); % 减小调整增益
    else % 如果误差在增大
        k_lambda = k_lambda * (1 + beta); % 增大调整增益
    end
    
    % 自适应调整k_eta
    if delta_de < 0 % 如果误差在减小
        k_eta = k_eta * (1 - alpha); % 减小调整增益
    else % 如果误差在增大
        k_eta = k_eta * (1 + beta); % 增大调整增益
    end
    
    % 自适应调整k_epsilon
    if delta_de < 0 % 如果误差在减小
        k_epsilon = k_epsilon * (1 - alpha); % 减小调整增益
    else % 如果误差在增大
        k_epsilon = k_epsilon * (1 + beta); % 增大调整增益
    end
    
    % 保证增益因子不为负数或过小
    k_lambda = max(k_lambda, 1e-3);
    k_eta = max(k_eta, 1e-3);
    k_epsilon = max(k_epsilon, 1e-3);
end
